simulink model "Buck_PWM"  (Simulink 10.0)
settings: Solver=ode45  StartTime=0.0  StopTime=4000.0  MaxStep=0.1  RelTol=1e-3  EnableMultiTasking=on
InitFcn:
  | buck1
undefined symbols (not defined in the file): C, L, RC, RL
libraries: simulink x4
settings Model: Creator=fo1521  LastModifiedBy=bhisma
settings DataIOCC: LimitDataPoints=on  SignalLoggingSaveFormat=ModelDataLogs
settings OptimizationCC: ExpressionDepthLimit=2147483647  InitFltsAndDblsToZero=on
settings DebuggingCC: SaveWithParameterizedLinksMsg=none  SignalResolutionControl=TryResolveAllWithWarning  SolverPrmCheckMsg=warning  MultiTaskDSMMsg=warning  MultiTaskCondExecSysMsg=none  FcnCallInpInsideContextMsg=warning  StateNameClashWarn=warning
settings SFSimCC: SimUseLocalCustomCode=on  CustomCodeUndefinedFunction=FilterOut
settings RTWCC: RTWUseLocalCustomCode=on
settings GRTTargetCC: TargetFcnLib=ansi_tfl_tmw.mat

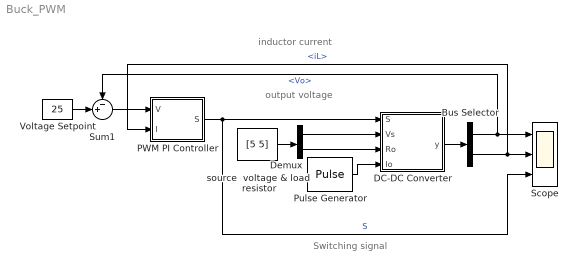
== system Buck_PWM ==
  note: Switching signal
  note: output voltage
  note: inductor current
  Bus Selector : BusSelector  OutputSignals=Vo,iL
  DC-DC Converter : Subsystem  mask{ICM=on, zcv=on, Vc0=0, ILmin=0, C=C, L=L, RC=RC, RL=RL, mode=Boost}
      mask prompts: ICM "Positive Inductor Current"; zcv "zero capacitor voltage"; mode "Converter Mode"
      mask help:
      | DC-DC Buck Convertor
      | C: Capacitance
      | L: Inductance
      | RC: Internal resistance of the capacitor
      | RL: Internal resistance of the inductor
      mask init:
      | dt=pi*0.3;
      | t1=0:0.1:pi+dt;t2=-dt:0.1:pi+dt;t3=[-dt:0.1:pi pi];
      | dx=2*cos(dt);
      | yL=5+[dx cos(t1)-1 cos(t2)-1-dx cos(t3)-1-2*dx -2-3*dx];
      | xL=[0 sin(t1) sin(t2) sin(t3) 0];
      | yC=[5+dx 2.5+dx NaN 2.5 0 NaN 2.5 2.5 NaN 2.5+dx 2.5+dx];
      | xC=3+[0    0    NaN  0      0 NaN -1     1      NaN -1     1];
      | x=[xL NaN xC NaN -3 NaN 6];
      | y=[yL NaN yC NaN -1 NaN 6];
      mask Callback ICM: converter_mask(gcb)
      mask Callback zcv: converter_mask(gcb)
      mask TypeOptions mode: Buck | Boost | Buck Boost
      mask Display:
      | plot(x,y)
      | port_label('output',1,'Y')
      | port_label('input',1,'S')
      | port_label('input',2,'Vi')
      | port_label('input',3,'Ro')
      | port_label('input',4,'Io')
  Demux : Demux  Outputs=2
  "PWM PI Controller " : Subsystem  mask{beta=0.2, Kp=1, Ti=300, Fs=0.2}
      mask help:
      | PWM PI Controller with Current Control
      | beta: gain for current control
      | Kp: Controller gain
      | Ti: Intergal time constant (s)
      | Fs: PWM frequency (Hz)
      mask Display: disp(sprintf('PWM PI\n Controller'))
  Pulse Generator : DiscretePulseGenerator  PulseType=Time based  Amplitude=0  PulseWidth=50
  Scope : Scope  NumInputPorts=3
  Sum1 : Sum  Inputs=-+|
  Voltage Setpoint : Constant  Value=25
  source  voltage & load  resistor : Constant  Value=[5 5]
  wires:
  "PWM PI Controller "/1(S) -> DC-DC Converter/1(S), Scope/3  "S"
  Bus Selector/1 -> Scope/1, Sum1/1  "<Vo>"
  source  voltage & load  resistor/1 -> Demux/1
  Demux/1 -> DC-DC Converter/2(Vs)
  Demux/2 -> DC-DC Converter/3(Ro)
  Pulse Generator/1 -> DC-DC Converter/4(Io)
  Bus Selector/2 -> Scope/2, "PWM PI Controller "/2(I)  "<iL>"
  DC-DC Converter/1(y) -> Bus Selector/1
  Sum1/1 -> "PWM PI Controller "/1(V)
  Voltage Setpoint/1 -> Sum1/2

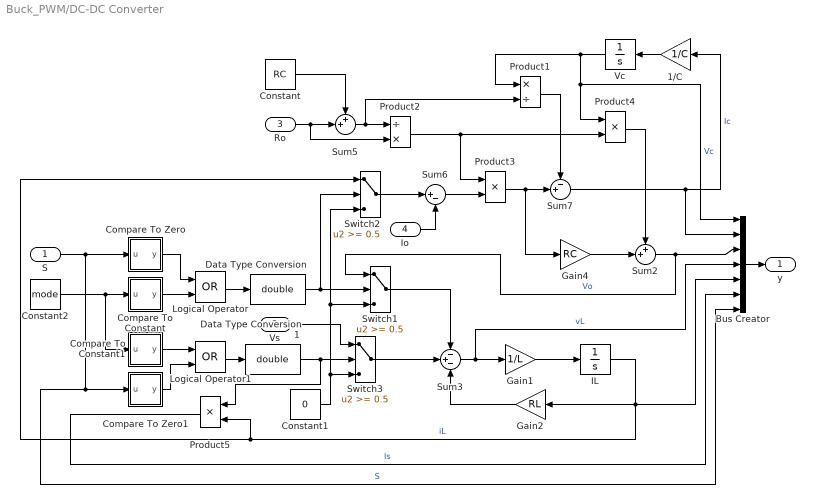
== system Buck_PWM/DC-DC Converter ==
  S : Inport
  Vs : Inport  Port=2
  Ro : Inport  Port=3
  Io : Inport  Port=4
  1/C : Gain  Gain=1/C  SaturateOnIntegerOverflow=on  OutDataTypeStr=Inherit: Same as input  ParamDataTypeStr=Inherit: Same as input
  Bus Creator : BusCreator  Inputs=7
  Compare To Constant : Subsystem  mask(Compare To Constant){relop===, const=1, LogicOutDataTypeMode=boolean}
      mask prompts: relop "Operator:"; const "Constant value:"; LogicOutDataTypeMode "Output data type mode:"
      mask help: Determine how a signal compares to a constant.
      mask init:
      | blkName = gcb;
      | 
      | if strcmp(get_param(gcbh,'LogicOutDataTypeMode'),'boolean')
      | 	setValue = 'Boolean';
      | else
      | 	setValue = 'Specify via dialog';
      | end
      | 
      | set_param([blkName,'/Compare'],'relop',relop, ...
      | 	'LogicOutDataTypeMode', setValue);
      | 
      | if length(const) == 1
      |  str = [relop,' ',num2str(double(const))];
      | else
      |   str = [relop,' C'];
      | end
      mask TypeOptions relop: == | ~= | < | <= | >= | >
      mask TypeOptions LogicOutDataTypeMode: uint8 | boolean
      mask Display: disp(str)
  Compare To Constant1 : Subsystem  mask(Compare To Constant){relop===, const=2, LogicOutDataTypeMode=boolean}
      mask prompts: relop "Operator:"; const "Constant value:"; LogicOutDataTypeMode "Output data type mode:"
      mask help: Determine how a signal compares to a constant.
      mask init: same as Buck_PWM/DC-DC Converter/Compare To Constant
      mask TypeOptions relop: == | ~= | < | <= | >= | >
      mask TypeOptions LogicOutDataTypeMode: uint8 | boolean
      mask Display: disp(str)
  Compare To Zero : Subsystem  mask(Compare To Zero){relop=>=, LogicOutDataTypeMode=boolean}
      mask prompts: relop "Operator:"; LogicOutDataTypeMode "Output data type mode:"
      mask help: Determine how a signal compares to zero.
      mask init:
      | blkName = gcb;
      | 
      | if strcmp(get_param(gcbh,'LogicOutDataTypeMode'),'boolean')
      | 	setValue = 'Boolean';
      | else
      |     setValue = 'Specify via dialog';
      | end
      | 
      | set_param([blkName,'/Compare'],'relop',relop, ...
      | 	'LogicOutDataTypeMode', setValue);
      mask TypeOptions relop: == | ~= | < | <= | >= | >
      mask TypeOptions LogicOutDataTypeMode: uint8 | boolean
      mask Display: disp([relop,' 0'])
  Compare To Zero1 : Subsystem  mask(Compare To Zero){relop=<, LogicOutDataTypeMode=boolean}
      mask prompts: relop "Operator:"; LogicOutDataTypeMode "Output data type mode:"
      mask help: Determine how a signal compares to zero.
      mask init: same as Buck_PWM/DC-DC Converter/Compare To Zero
      mask TypeOptions relop: == | ~= | < | <= | >= | >
      mask TypeOptions LogicOutDataTypeMode: uint8 | boolean
      mask Display: disp([relop,' 0'])
  Constant : Constant  Value=RC
  Constant1 : Constant  Value=0
  Constant2 : Constant  Value=mode
  Data Type Conversion : DataTypeConversion  OutDataTypeStr=double
  Data Type Conversion1 : DataTypeConversion  OutDataTypeStr=double
  Gain1 : Gain  Gain=1/L  SaturateOnIntegerOverflow=on  OutDataTypeStr=Inherit: Same as input  ParamDataTypeStr=Inherit: Same as input
  Gain2 : Gain  Gain=RL  SaturateOnIntegerOverflow=on  OutDataTypeStr=Inherit: Same as input  ParamDataTypeStr=Inherit: Same as input
  Gain4 : Gain  Gain=RC  SaturateOnIntegerOverflow=on  OutDataTypeStr=Inherit: Same as input  ParamDataTypeStr=Inherit: Same as input
  IL : Integrator  LimitOutput=on  LowerSaturationLimit=0
  Logical Operator : Logic  Operator=OR  AllPortsSameDT=off  OutDataTypeStr=boolean
  Logical Operator1 : Logic  Operator=OR  AllPortsSameDT=off  OutDataTypeStr=boolean
  Product1 : Product  Inputs=*/  SaturateOnIntegerOverflow=on  OutDataTypeStr=Inherit: Same as first input
  Product2 : Product  Inputs=/*  SaturateOnIntegerOverflow=on  OutDataTypeStr=Inherit: Same as first input
  Product3 : Product  SaturateOnIntegerOverflow=on  OutDataTypeStr=Inherit: Same as first input
  Product4 : Product  SaturateOnIntegerOverflow=on  OutDataTypeStr=Inherit: Same as first input
  Product5 : Product  SaturateOnIntegerOverflow=on  OutDataTypeStr=Inherit: Same as first input
  Sum2 : Sum  Inputs=++|  SaturateOnIntegerOverflow=on
  Sum3 : Sum  Inputs=-+-  SaturateOnIntegerOverflow=on
  Sum5 : Sum  Inputs=++|  SaturateOnIntegerOverflow=on
  Sum6 : Sum  Inputs=|+-  SaturateOnIntegerOverflow=on
  Sum7 : Sum  Inputs=-+|  SaturateOnIntegerOverflow=on
  Switch1 : Switch  Threshold=0.5  SaturateOnIntegerOverflow=on
  Switch2 : Switch  Threshold=0.5  SaturateOnIntegerOverflow=on
  Switch3 : Switch  Threshold=0.5  SaturateOnIntegerOverflow=on
  Vc : Integrator
  y : Outport
  wires:
  Bus Creator/1 -> y/1
  Data Type Conversion1/1 -> Switch3/2, Product5/1
  Data Type Conversion/1 -> Switch1/2, Switch2/2
  Gain1/1 -> IL/1
  Sum3/1 -> Bus Creator/4, Gain1/1  "vL"
  IL/1 -> Bus Creator/5, Gain2/1, Switch2/1, Product5/2  "iL"
  Ro/1 -> Sum5/2, Product2/2
  Constant/1 -> Sum5/1
  Gain2/1 -> Sum3/3
  Switch3/1 -> Sum3/2
  Switch1/1 -> Sum3/1
  Logical Operator/1 -> Data Type Conversion/1
  Constant1/1 -> Switch3/3, Switch1/3, Switch2/3
  Vs/1 -> Switch3/1
  Logical Operator1/1 -> Data Type Conversion1/1
  Switch2/1 -> Sum6/1
  Io/1 -> Sum6/2
  Sum5/1 -> Product2/1, Product1/2
  Sum6/1 -> Product3/2
  Product2/1 -> Product3/1, Product4/2
  Product3/1 -> Sum7/2, Gain4/1
  Sum7/1 -> Bus Creator/2, 1/C/1  "Ic"
  Product1/1 -> Sum7/1
  Gain4/1 -> Sum2/2
  Product4/1 -> Sum2/1
  Sum2/1 -> Bus Creator/3, Switch1/1  "Vo"
  Constant2/1 -> Compare To Constant/1(u), Compare To Constant1/1(u)
  S/1 -> Bus Creator/7, Compare To Zero1/1(u), Compare To Zero/1(u)  "S"
  Compare To Zero/1(y) -> Logical Operator/1
  Compare To Constant/1(y) -> Logical Operator/2
  Compare To Zero1/1(y) -> Logical Operator1/2
  Compare To Constant1/1(y) -> Logical Operator1/1
  Product5/1 -> Bus Creator/6  "Is"
  Vc/1 -> Bus Creator/1, Product4/1, Product1/1  "Vc"
  1/C/1 -> Vc/1

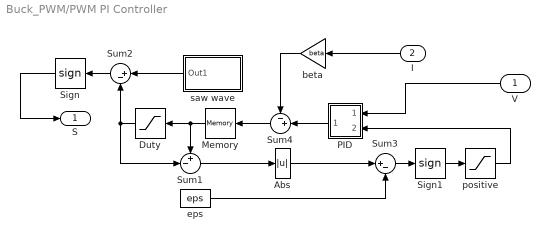
== system Buck_PWM/PWM PI Controller  ==
  V : Inport
  I : Inport  Port=2
  Abs : Abs
  Duty : Saturate  UpperLimit=0.99  LowerLimit=0.01
  Memory : Memory
  PID : Subsystem  mask(PID Controller){P=Kp, I=Kp/Ti, D=0}
      mask prompts: P "Proportional:"; I "Integral:"; D "Derivative:"
      mask help:
      | Enter expressions for proportional, integral, and derivative terms.
      | P+I/s+Ds
      mask Help: This block implements a PID controller where parameters are entered for the Proportional, Integral and Derivative terms. Unmask this block to see how it works. The derivative term is implemented using a true derivative block.
      mask Display: disp('PID')
  Sign : Signum
  Sign1 : Signum
  Sum1 : Sum  Inputs=+-|
  Sum2 : Sum  Inputs=|+-
  Sum3 : Sum  Inputs=|+-
  Sum4 : Sum  Inputs=-+|
  beta : Gain  Gain=beta
  eps : Constant  Value=eps
  positive : Saturate  UpperLimit=1  LowerLimit=0
  saw wave : Subsystem  mask{fs=Fs}
      mask init:
      | x=[-1 NaN 4 NaN 0 1 1 2 2 3 3];
      | y=[-0.5 NaN 1.5 NaN 0 1 0 1 0 1 0];
      mask Display:
      | plot(x,y);
      | port_label('output',1,'S')
  S : Outport
  wires:
  Duty/1 -> Sum2/2, Sum1/2
  saw wave/1(Out1) -> Sum2/1
  Sum2/1 -> Sign/1
  Sign/1 -> S/1
  Sign1/1 -> positive/1
  Sum1/1 -> Abs/1
  Abs/1 -> Sum3/1
  Sum3/1 -> Sign1/1
  eps/1 -> Sum3/2
  I/1 -> beta/1
  positive/1 -> PID/2(In_2)
  beta/1 -> Sum4/1
  Memory/1 -> Duty/1, Sum1/1
  Sum4/1 -> Memory/1
  V/1 -> PID/1(In_1)
  PID/1(Out_1) -> Sum4/2

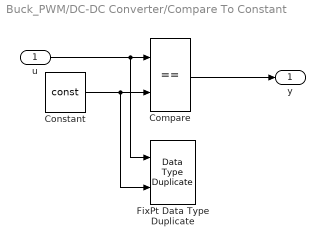
== system Buck_PWM/DC-DC Converter/Compare To Constant ==
  u : Inport
  Compare : RelationalOperator  Operator===  OutDataTypeStr=boolean  ZeroCross=off  RndMeth=Nearest
  Constant : Constant  Value=const  OutDataTypeStr=Inherit: Inherit via back propagation
  FixPt Data Type Duplicate : simulink/Signal Attributes/Data Type Duplicate  NumInputPorts=2
      settings: SourceProductName=Simulink  SourceProductBaseCode=SL
  y : Outport
  wires:
  u/1 -> Compare/1, FixPt Data Type Duplicate/1
  Constant/1 -> Compare/2, FixPt Data Type Duplicate/2
  Compare/1 -> y/1

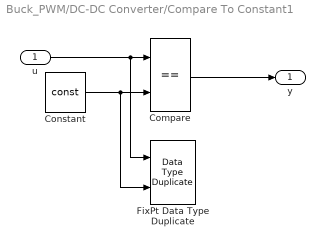
== system Buck_PWM/DC-DC Converter/Compare To Constant1 ==
  u : Inport
  Compare : RelationalOperator  Operator===  OutDataTypeStr=boolean  ZeroCross=off  RndMeth=Nearest
  Constant : Constant  Value=const  OutDataTypeStr=Inherit: Inherit via back propagation
  FixPt Data Type Duplicate : simulink/Signal Attributes/Data Type Duplicate  NumInputPorts=2
      settings: SourceProductName=Simulink  SourceProductBaseCode=SL
  y : Outport
  wires:
  Compare/1 -> y/1
  Constant/1 -> FixPt Data Type Duplicate/2, Compare/2
  u/1 -> FixPt Data Type Duplicate/1, Compare/1

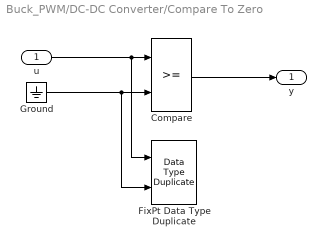
== system Buck_PWM/DC-DC Converter/Compare To Zero ==
  u : Inport
  Compare : RelationalOperator  OutDataTypeStr=boolean  ZeroCross=off  RndMeth=Nearest
  FixPt Data Type Duplicate : simulink/Signal Attributes/Data Type Duplicate  NumInputPorts=2
      settings: SourceProductName=Simulink  SourceProductBaseCode=SL
  Ground : Ground
  y : Outport
  wires:
  u/1 -> Compare/1, FixPt Data Type Duplicate/1
  Ground/1 -> Compare/2, FixPt Data Type Duplicate/2
  Compare/1 -> y/1

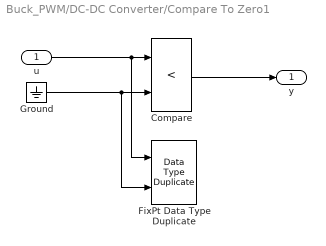
== system Buck_PWM/DC-DC Converter/Compare To Zero1 ==
  u : Inport
  Compare : RelationalOperator  Operator=<  OutDataTypeStr=boolean  ZeroCross=off  RndMeth=Nearest
  FixPt Data Type Duplicate : simulink/Signal Attributes/Data Type Duplicate  NumInputPorts=2
      settings: SourceProductName=Simulink  SourceProductBaseCode=SL
  Ground : Ground
  y : Outport
  wires:
  Compare/1 -> y/1
  Ground/1 -> FixPt Data Type Duplicate/2, Compare/2
  u/1 -> FixPt Data Type Duplicate/1, Compare/1

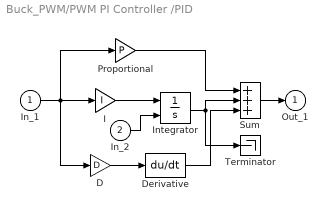
== system Buck_PWM/PWM PI Controller /PID ==
  In_1 : Inport
  In_2 : Inport  Port=2
  D : Gain  Gain=D  SaturateOnIntegerOverflow=on  OutDataTypeStr=Inherit: Same as input  ParamDataTypeStr=Inherit: Same as input
  Derivative : Derivative
  I : Gain  Gain=I  SaturateOnIntegerOverflow=on  OutDataTypeStr=Inherit: Same as input  ParamDataTypeStr=Inherit: Same as input
  Integrator : Integrator  ExternalReset=level
  Proportional : Gain  Gain=P  SaturateOnIntegerOverflow=on  OutDataTypeStr=Inherit: Same as input  ParamDataTypeStr=Inherit: Same as input
  Sum : Sum  Inputs=+++  SaturateOnIntegerOverflow=on  InputSameDT=on  OutDataTypeStr=Inherit: Same as first input
  Terminator : Terminator
  Out_1 : Outport  InitialOutput=0
  wires:
  Integrator/1 -> Sum/2, Terminator/1
  Proportional/1 -> Sum/1
  Derivative/1 -> Sum/3
  In_1/1 -> Proportional/1, I/1, D/1
  Sum/1 -> Out_1/1
  D/1 -> Derivative/1
  I/1 -> Integrator/1
  In_2/1 -> Integrator/2

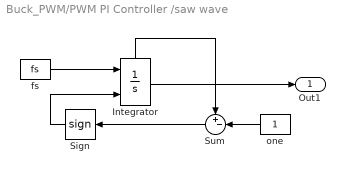
== system Buck_PWM/PWM PI Controller /saw wave ==
  Integrator : Integrator  ExternalReset=rising  ShowStatePort=on
  Sign : Signum
  Sum : Sum  Inputs=+-|
  fs : Constant  Value=fs
  one : Constant
  Out1 : Outport
  wires:
  Integrator/1 -> Out1/1
  Sum/1 -> Sign/1
  fs/1 -> Integrator/1
  one/1 -> Sum/2
  Sign/1 -> Integrator/2
  Integrator/State -> Sum/1
